simulink model "PA11_13_sim"  (R2024a)
settings: Solver=ode4  StartTime=0.0  StopTime=10.0  FixedStep=0.01  RelTol=1e-3
values from neighbouring files (symbols this model uses):
  A = [1, 2; -6, -12]    [PA11_13.m]
  B = [-5; 1]    [PA11_13.m]
  C = [4, -3]    [PA11_13.m]
  K = acker(A, B, p)    [PA11_13.m]
  Ke = acker(ss_dual.A, ss_dual.B, po')'    [PA11_13.m]
  x0 = [1;2]    [PA11_13.m]
  x0_o = [1;0]    [PA11_13.m]
settings Model: Creator=caugu  LastModifiedBy=caugu

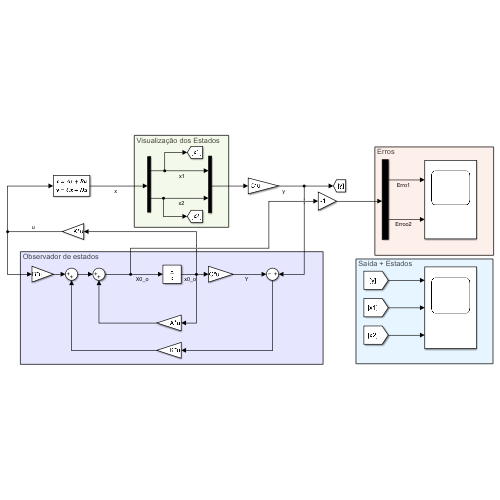
[thumbnail: Simulink's stored preview of the top-level diagram]
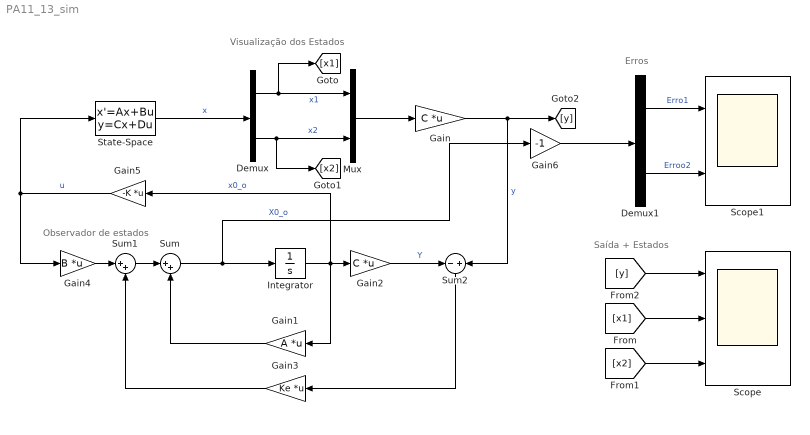
== system PA11_13_sim ==
  note: Visualização dos Estados
  note: Erros
  note: Saída + Estados
  note: Observador de estados
  Demux : Demux  Outputs=2
  Demux1 : Demux  Outputs=2
  Gain : Gain  Gain=C  Multiplication=Matrix(K*u)
  Gain1 : Gain  Gain=A  Multiplication=Matrix(K*u)
  Gain2 : Gain  Gain=C  Multiplication=Matrix(K*u)
  Gain3 : Gain  Gain=Ke  Multiplication=Matrix(K*u)
  Gain4 : Gain  Gain=B  Multiplication=Matrix(K*u)
  Gain5 : Gain  Gain=-K  Multiplication=Matrix(K*u)
  Gain6 : Gain  Gain=-1
  Integrator : Integrator  InitialCondition=x0_o
  Mux : Mux  Inputs=2
  Scope : Scope  NumInputPorts=3
  Scope1 : Scope  NumInputPorts=2
  State-Space : StateSpace  A=A  B=B  C=eye(2)  D=zeros(2,1)  InitialCondition=x0
  Sum : Sum  Inputs=|++
  Sum1 : Sum  Inputs=|++
  Sum2 : Sum  Inputs=-+
  wires:
  Demux1/1 -> Scope1/1  "Erro1"
  Sum/1 -> Gain6/1, Integrator/1  "X0_o"
  Demux/1 -> [x1], Mux/1  "x1"
  Gain6/1 -> Demux1/1
  Gain/1 -> [y], Sum2/2  "y"
  Mux/1 -> Gain/1
  [x1] -> Scope/2
  [y] -> Scope/1
  State-Space/1 -> Demux/1  "x"
  Integrator/1 -> Gain5/1, Gain2/1, Gain1/1  "x0_o"
  Sum1/1 -> Sum/1
  Demux/2 -> [x2], Mux/2  "x2"
  Sum2/1 -> Gain3/1
  Gain2/1 -> Sum2/1  "Y"
  Gain4/1 -> Sum1/1
  Gain1/1 -> Sum/2
  Gain5/1 -> State-Space/1, Gain4/1  "u"
  Demux1/2 -> Scope1/2  "Erroo2"
  Gain3/1 -> Sum1/2
  [x2] -> Scope/3
